simulink subsystem "PowerSystemRef"  (R2024b)
settings: Solver=VariableStepAuto  StartTime=0.0  StopTime=10.0  RelTol=1e-3
undefined symbols (not defined in the file): ess, geom, mot, mot2, mot3, mot4, propel, propel2, propel3, propel4, pxf_diagram_options, SimIn, tc, tc2, tc3, tc4
libraries: simulink x10, slpidlib x5
(part 4 of 10)

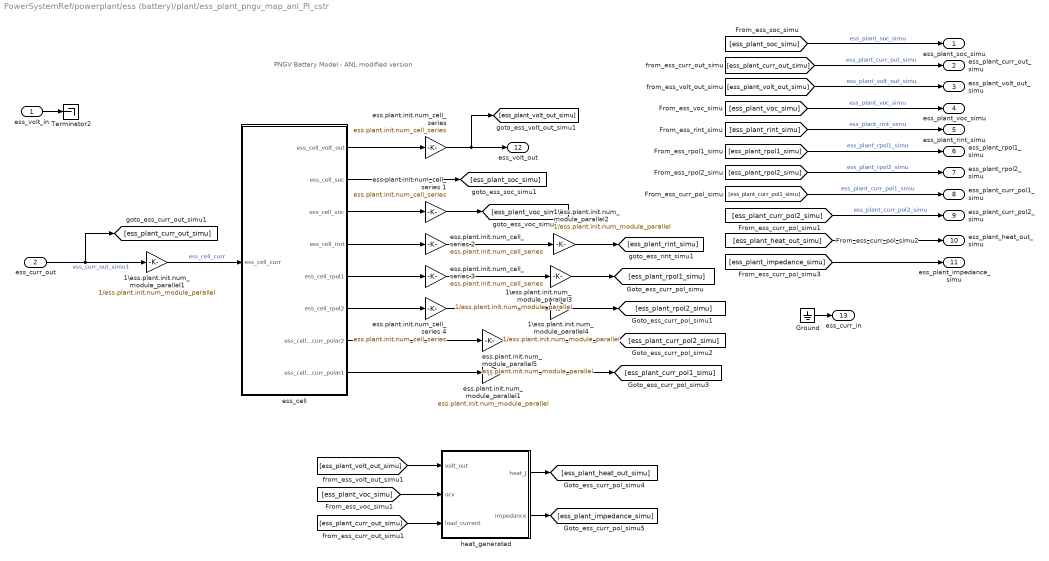
== system PowerSystemRef/powerplant/ess (battery)/plant/ess_plant_pngv_map_anl_PI_cstr ==
  note: PNGV Battery Model - ANL modified version
  ess_volt_in : Inport
  ess_curr_out : Inport  Port=2
  1\ess.plant.init.num_module_parallel{1..4} (4 alike) : Gain  Gain=1/ess.plant.init.num_module_parallel
  Ground : Ground
  Terminator2 : Terminator
  ess.plant.init.num_cell_series {,1..4} (5 alike) : Gain  Gain=ess.plant.init.num_cell_series
  ess.plant.init.num_module_parallel1 : Gain  Gain=ess.plant.init.num_module_parallel
  ess.plant.init.num_module_parallel5 : Gain  Gain=ess.plant.init.num_module_parallel
  ess_cell : Subsystem
  heat_generated : Subsystem
  ess_plant_soc_simu : Outport
  ess_plant_curr_out_simu : Outport  Port=2
  ess_plant_volt_out_simu : Outport  Port=3
  ess_plant_voc_simu : Outport  Port=4
  ess_plant_rint_simu : Outport  Port=5
  ess_plant_rpol1_simu : Outport  Port=6
  ess_plant_rpol2_simu : Outport  Port=7
  ess_plant_curr_pol1_simu : Outport  Port=8
  ess_plant_curr_pol2_simu : Outport  Port=9
  ess_plant_heat_out_simu : Outport  Port=10
  ess_plant_impedance_simu : Outport  Port=11
  ess_volt_out : Outport  Port=12
  ess_curr_in : Outport  Port=13
  wires:
  [ess_plant_impedance_simu] -> ess_plant_impedance_simu/1
  heat_generated/2(impedance) -> [ess_plant_impedance_simu]
  [ess_plant_heat_out_simu] -> ess_plant_heat_out_simu/1
  heat_generated/1(heat_J) -> [ess_plant_heat_out_simu]
  [ess_plant_curr_out_simu] -> heat_generated/3(load_current)
  [ess_plant_voc_simu] -> heat_generated/2(ocv)
  [ess_plant_volt_out_simu] -> heat_generated/1(volt_out)
  ess.plant.init.num_module_parallel1/1 -> [ess_plant_curr_pol1_simu]
  ess.plant.init.num_module_parallel5/1 -> [ess_plant_curr_pol2_simu]
  ess_cell/7(ess_cell_curr_polar2) -> ess.plant.init.num_module_parallel5/1
  ess_cell/8(ess_cell_curr_polar1) -> ess.plant.init.num_module_parallel1/1
  1\ess.plant.init.num_module_parallel4/1 -> [ess_plant_rpol2_simu]
  ess.plant.init.num_cell_series 4/1 -> 1\ess.plant.init.num_module_parallel4/1
  1\ess.plant.init.num_module_parallel3/1 -> [ess_plant_rpol1_simu]
  ess.plant.init.num_cell_series 3/1 -> 1\ess.plant.init.num_module_parallel3/1
  ess_cell/6(ess_cell_rpol2) -> ess.plant.init.num_cell_series 4/1
  ess_cell/5(ess_cell_rpol1) -> ess.plant.init.num_cell_series 3/1
  ess_cell/2(ess_cell_soc) -> [ess_plant_soc_simu]
  ess_cell/4(ess_cell_rint) -> ess.plant.init.num_cell_series 2/1
  ess_cell/3(ess_cell_voc) -> ess.plant.init.num_cell_series 1/1
  ess_curr_out/1 -> [ess_plant_curr_out_simu], 1\ess.plant.init.num_module_parallel1/1  "ess_curr_out_simu1"
  1\ess.plant.init.num_module_parallel2/1 -> [ess_plant_rint_simu]
  ess.plant.init.num_cell_series 1/1 -> [ess_plant_voc_simu]
  ess.plant.init.num_cell_series 2/1 -> 1\ess.plant.init.num_module_parallel2/1
  "ess.plant.init.num_cell_series "/1 -> ess_volt_out/1, [ess_plant_volt_out_simu]
  1\ess.plant.init.num_module_parallel1/1 -> ess_cell/1(ess_cell_curr)  "ess_cell_curr"
  ess_cell/1(ess_cell_volt_out) -> "ess.plant.init.num_cell_series "/1
  [ess_plant_curr_pol2_simu] -> ess_plant_curr_pol2_simu/1  "ess_plant_curr_pol2_simu"
  [ess_plant_curr_pol1_simu] -> ess_plant_curr_pol1_simu/1  "ess_plant_curr_pol1_simu"
  [ess_plant_rpol2_simu] -> ess_plant_rpol2_simu/1  "ess_plant_rpol2_simu"
  [ess_plant_rpol1_simu] -> ess_plant_rpol1_simu/1  "ess_plant_rpol1_simu"
  [ess_plant_rint_simu] -> ess_plant_rint_simu/1  "ess_plant_rint_simu"
  [ess_plant_voc_simu] -> ess_plant_voc_simu/1  "ess_plant_voc_simu"
  [ess_plant_volt_out_simu] -> ess_plant_volt_out_simu/1  "ess_plant_volt_out_simu"
  [ess_plant_curr_out_simu] -> ess_plant_curr_out_simu/1  "ess_plant_curr_out_simu"
  [ess_plant_soc_simu] -> ess_plant_soc_simu/1  "ess_plant_soc_simu"
  ess_volt_in/1 -> Terminator2/1
  Ground/1 -> ess_curr_in/1

== system PowerSystemRef/powerplant/ess (battery)/plant/parameter_out ==
  inport-ess_plant_soc_simu : Inport
  inport-ess_plant_curr_out_simu : Inport  Port=2
  inport-ess_plant_volt_out_simu : Inport  Port=3
  inport-ess_plant_voc_simu : Inport  Port=4
  inport-ess_plant_rint_simu : Inport  Port=5
  inport-ess_plant_rpol1_simu : Inport  Port=6
  inport-ess_plant_rpol2_simu : Inport  Port=7
  inport-ess_plant_curr_pol1_simu : Inport  Port=8
  inport-ess_plant_curr_pol2_simu : Inport  Port=9
  inport-ess_plant_heat_out_simu : Inport  Port=10
  inport-ess_plant_impedance_simu : Inport  Port=11
  Ground_1 : Ground
  Toworkspace-ess_plant_curr_out_simu : ToWorkspace  VariableName=ess_plant_curr_out_simu  SampleTime=pxf_diagram_options.workspace_sample_time
      settings: Decimation=pxf_diagram_options.decimation
  Toworkspace-ess_plant_curr_pol1_simu : ToWorkspace  VariableName=ess_plant_curr_pol1_simu  SampleTime=pxf_diagram_options.workspace_sample_time
      settings: Decimation=pxf_diagram_options.decimation
  Toworkspace-ess_plant_curr_pol2_simu : ToWorkspace  VariableName=ess_plant_curr_pol2_simu  SampleTime=pxf_diagram_options.workspace_sample_time
      settings: Decimation=pxf_diagram_options.decimation
  Toworkspace-ess_plant_heat_out_simu : ToWorkspace  VariableName=ess_plant_heat_out_simu  SampleTime=pxf_diagram_options.workspace_sample_time
      settings: Decimation=pxf_diagram_options.decimation
  Toworkspace-ess_plant_impedance_simu : ToWorkspace  VariableName=ess_plant_impedance_simu  SampleTime=pxf_diagram_options.workspace_sample_time
      settings: Decimation=pxf_diagram_options.decimation
  Toworkspace-ess_plant_rint_simu : ToWorkspace  VariableName=ess_plant_rint_simu  SampleTime=pxf_diagram_options.workspace_sample_time
      settings: Decimation=pxf_diagram_options.decimation
  Toworkspace-ess_plant_rpol1_simu : ToWorkspace  VariableName=ess_plant_rpol1_simu  SampleTime=pxf_diagram_options.workspace_sample_time
      settings: Decimation=pxf_diagram_options.decimation
  Toworkspace-ess_plant_rpol2_simu : ToWorkspace  VariableName=ess_plant_rpol2_simu  SampleTime=pxf_diagram_options.workspace_sample_time
      settings: Decimation=pxf_diagram_options.decimation
  Toworkspace-ess_plant_soc_simu : ToWorkspace  VariableName=ess_plant_soc_simu  SampleTime=pxf_diagram_options.workspace_sample_time
      settings: Decimation=pxf_diagram_options.decimation
  Toworkspace-ess_plant_voc_simu : ToWorkspace  VariableName=ess_plant_voc_simu  SampleTime=pxf_diagram_options.workspace_sample_time
      settings: Decimation=pxf_diagram_options.decimation
  Toworkspace-ess_plant_volt_out_simu : ToWorkspace  VariableName=ess_plant_volt_out_simu  SampleTime=pxf_diagram_options.workspace_sample_time
      settings: Decimation=pxf_diagram_options.decimation
  create_system_info_bus : BusCreator  Inputs=3
  outport-system_info_bus : Outport
  outport-plant_bus : Outport  Port=2
  wires:
  create_system_info_bus/1 -> outport-system_info_bus/1
  inport-ess_plant_soc_simu/1 -> create_system_info_bus/1, Toworkspace-ess_plant_soc_simu/1  "ess_plant_soc_simu"
  inport-ess_plant_heat_out_simu/1 -> Toworkspace-ess_plant_heat_out_simu/1
  inport-ess_plant_impedance_simu/1 -> Toworkspace-ess_plant_impedance_simu/1
  inport-ess_plant_curr_out_simu/1 -> create_system_info_bus/2, Toworkspace-ess_plant_curr_out_simu/1  "ess_plant_curr_out_simu"
  inport-ess_plant_volt_out_simu/1 -> create_system_info_bus/3, Toworkspace-ess_plant_volt_out_simu/1  "ess_plant_volt_out_simu"
  inport-ess_plant_voc_simu/1 -> Toworkspace-ess_plant_voc_simu/1
  inport-ess_plant_rint_simu/1 -> Toworkspace-ess_plant_rint_simu/1
  inport-ess_plant_rpol1_simu/1 -> Toworkspace-ess_plant_rpol1_simu/1
  inport-ess_plant_rpol2_simu/1 -> Toworkspace-ess_plant_rpol2_simu/1
  inport-ess_plant_curr_pol1_simu/1 -> Toworkspace-ess_plant_curr_pol1_simu/1
  inport-ess_plant_curr_pol2_simu/1 -> Toworkspace-ess_plant_curr_pol2_simu/1
  Ground_1/1 -> outport-plant_bus/1

== system PowerSystemRef/powerplant/ess (battery)/plant/parameter_selection ==

== system PowerSystemRef/powerplant/ess (battery)1/ctrl/ess_ctrl_pngv_map_anl_PI_cstr ==
  ess_volt_out : Inport
  ess_curr_out : Inport  Port=2
  ess_soc : Inport  Port=3
  Demux : Demux  Outputs=3
  Demux1 : Demux  Outputs=3
  PI controller for maximal charge power and current1 : Subsystem
  PI controller for maximal discharge power and current1 : Subsystem
  mux1 : Mux  Inputs=3
  ess_ctrl_pwr_max_pro_simu : Outport
  ess_ctrl_pwr_max_reg_simu : Outport  Port=2
  ess_ctrl_curr_max_pro_simu : Outport  Port=3
  ess_ctrl_curr_max_reg_simu : Outport  Port=4
  wires:
  [ess_ctrl_pwr_max_reg_simu] -> ess_ctrl_pwr_max_reg_simu/1  "ess_ctrl_pwr_max_reg_simu"
  [ess_ctrl_pwr_max_pro_simu] -> ess_ctrl_pwr_max_pro_simu/1  "ess_ctrl_pwr_max_pro_simu"
  [ess_ctrl_curr_max_pro_simu] -> ess_ctrl_curr_max_pro_simu/1  "ess_ctrl_curr_max_pro_simu"
  [ess_ctrl_curr_max_reg_simu] -> ess_ctrl_curr_max_reg_simu/1  "ess_ctrl_curr_max_reg_simu"
  PI controller for maximal discharge power and current1/1(Curr_max_prop) -> [ess_ctrl_curr_max_pro_simu]
  PI controller for maximal charge power and current1/2(Curr_max_reg) -> [ess_ctrl_curr_max_reg_simu]
  ess_volt_out/1 -> mux1/1  "ess_plant_volt_out_simu"
  mux1/1 -> Demux/1, Demux1/1
  PI controller for maximal discharge power and current1/2(Pwr_max_prop) -> [ess_ctrl_pwr_max_pro_simu]
  PI controller for maximal charge power and current1/1(Pwr_max_reg) -> [ess_ctrl_pwr_max_reg_simu]
  Demux/1 -> PI controller for maximal discharge power and current1/1(ess voltage)
  Demux/2 -> PI controller for maximal discharge power and current1/2(ess curr)
  Demux/3 -> PI controller for maximal discharge power and current1/3(SOC)
  Demux1/1 -> PI controller for maximal charge power and current1/1(ess voltage)
  Demux1/2 -> PI controller for maximal charge power and current1/2(ess curr)
  Demux1/3 -> PI controller for maximal charge power and current1/3(SOC)
  ess_curr_out/1 -> mux1/2  "ess_plant_curr_out_simu"
  ess_soc/1 -> mux1/3  "ess_plant_soc_simu"

== system PowerSystemRef/powerplant/ess (battery)1/ctrl/parameter_out ==
  inport-ess_ctrl_pwr_max_pro_simu : Inport
  inport-ess_ctrl_pwr_max_reg_simu : Inport  Port=2
  inport-ess_ctrl_curr_max_pro_simu : Inport  Port=3
  inport-ess_ctrl_curr_max_reg_simu : Inport  Port=4
  Ground_1 : Ground
  Toworkspace-ess_ctrl_curr_max_pro_simu : ToWorkspace  VariableName=ess_ctrl_curr_max_pro_simu  SampleTime=pxf_diagram_options.workspace_sample_time
      settings: Decimation=pxf_diagram_options.decimation
  Toworkspace-ess_ctrl_curr_max_reg_simu : ToWorkspace  VariableName=ess_ctrl_curr_max_reg_simu  SampleTime=pxf_diagram_options.workspace_sample_time
      settings: Decimation=pxf_diagram_options.decimation
  Toworkspace-ess_ctrl_pwr_max_pro_simu : ToWorkspace  VariableName=ess_ctrl_pwr_max_pro_simu  SampleTime=pxf_diagram_options.workspace_sample_time
      settings: Decimation=pxf_diagram_options.decimation
  Toworkspace-ess_ctrl_pwr_max_reg_simu : ToWorkspace  VariableName=ess_ctrl_pwr_max_reg_simu  SampleTime=pxf_diagram_options.workspace_sample_time
      settings: Decimation=pxf_diagram_options.decimation
  create_system_info_bus : BusCreator  Inputs=1
  outport-system_info_bus : Outport
  outport-ctrl_bus : Outport  Port=2
  wires:
  Ground_1/1 -> outport-ctrl_bus/1
  inport-ess_ctrl_curr_max_reg_simu/1 -> Toworkspace-ess_ctrl_curr_max_reg_simu/1
  inport-ess_ctrl_curr_max_pro_simu/1 -> Toworkspace-ess_ctrl_curr_max_pro_simu/1
  inport-ess_ctrl_pwr_max_reg_simu/1 -> Toworkspace-ess_ctrl_pwr_max_reg_simu/1
  inport-ess_ctrl_pwr_max_pro_simu/1 -> Toworkspace-ess_ctrl_pwr_max_pro_simu/1, create_system_info_bus/1  "ess_ctrl_pwr_max_pro_simu"
  create_system_info_bus/1 -> outport-system_info_bus/1

== system PowerSystemRef/powerplant/ess (battery)1/ctrl/parameter_selection ==
  inport-main_info_bus-1 : Inport
  select_main_info_bus : BusSelector  OutputSignals=apa_info_bus.powerplant_info_bus.ess.plant.ess_plant_volt_out_simu,apa_info_bus.powerplant_info_bus.ess.plant.ess_plant_curr_out_simu,apa_info_bus.powerplant_info_bus.ess.plant.ess_plant_soc_simu
  outport-ess_plant_volt_out_simu-1 : Outport
  outport-ess_plant_curr_out_simu-2 : Outport  Port=2
  outport-ess_plant_soc_simu-3 : Outport  Port=3
  wires:
  select_main_info_bus/3 -> outport-ess_plant_soc_simu-3/1  "<ess_plant_soc_simu>"
  select_main_info_bus/2 -> outport-ess_plant_curr_out_simu-2/1  "<ess_plant_curr_out_simu>"
  select_main_info_bus/1 -> outport-ess_plant_volt_out_simu-1/1  "<ess_plant_volt_out_simu>"
  inport-main_info_bus-1/1 -> select_main_info_bus/1

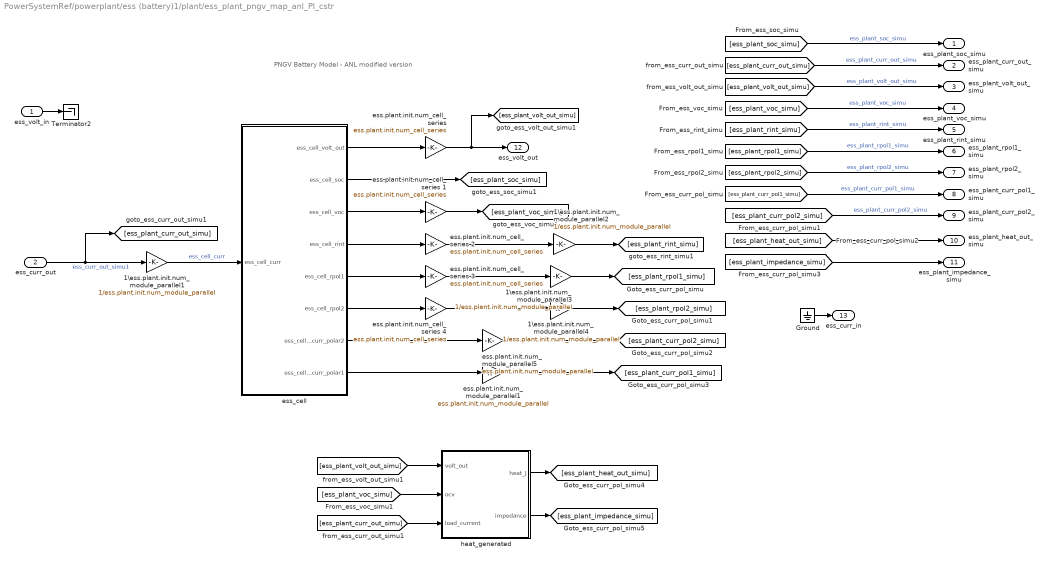
== system PowerSystemRef/powerplant/ess (battery)1/plant/ess_plant_pngv_map_anl_PI_cstr ==
  note: PNGV Battery Model - ANL modified version
  ess_volt_in : Inport
  ess_curr_out : Inport  Port=2
  1\ess.plant.init.num_module_parallel{1..4} (4 alike) : Gain  Gain=1/ess.plant.init.num_module_parallel
  Ground : Ground
  Terminator2 : Terminator
  ess.plant.init.num_cell_series {,1..4} (5 alike) : Gain  Gain=ess.plant.init.num_cell_series
  ess.plant.init.num_module_parallel1 : Gain  Gain=ess.plant.init.num_module_parallel
  ess.plant.init.num_module_parallel5 : Gain  Gain=ess.plant.init.num_module_parallel
  ess_cell : Subsystem
  heat_generated : Subsystem
  ess_plant_soc_simu : Outport
  ess_plant_curr_out_simu : Outport  Port=2
  ess_plant_volt_out_simu : Outport  Port=3
  ess_plant_voc_simu : Outport  Port=4
  ess_plant_rint_simu : Outport  Port=5
  ess_plant_rpol1_simu : Outport  Port=6
  ess_plant_rpol2_simu : Outport  Port=7
  ess_plant_curr_pol1_simu : Outport  Port=8
  ess_plant_curr_pol2_simu : Outport  Port=9
  ess_plant_heat_out_simu : Outport  Port=10
  ess_plant_impedance_simu : Outport  Port=11
  ess_volt_out : Outport  Port=12
  ess_curr_in : Outport  Port=13
  wires:
  Ground/1 -> ess_curr_in/1
  ess_volt_in/1 -> Terminator2/1
  [ess_plant_soc_simu] -> ess_plant_soc_simu/1  "ess_plant_soc_simu"
  [ess_plant_curr_out_simu] -> ess_plant_curr_out_simu/1  "ess_plant_curr_out_simu"
  [ess_plant_volt_out_simu] -> ess_plant_volt_out_simu/1  "ess_plant_volt_out_simu"
  [ess_plant_voc_simu] -> ess_plant_voc_simu/1  "ess_plant_voc_simu"
  [ess_plant_rint_simu] -> ess_plant_rint_simu/1  "ess_plant_rint_simu"
  [ess_plant_rpol1_simu] -> ess_plant_rpol1_simu/1  "ess_plant_rpol1_simu"
  [ess_plant_rpol2_simu] -> ess_plant_rpol2_simu/1  "ess_plant_rpol2_simu"
  [ess_plant_curr_pol1_simu] -> ess_plant_curr_pol1_simu/1  "ess_plant_curr_pol1_simu"
  [ess_plant_curr_pol2_simu] -> ess_plant_curr_pol2_simu/1  "ess_plant_curr_pol2_simu"
  ess_cell/1(ess_cell_volt_out) -> "ess.plant.init.num_cell_series "/1
  1\ess.plant.init.num_module_parallel1/1 -> ess_cell/1(ess_cell_curr)  "ess_cell_curr"
  "ess.plant.init.num_cell_series "/1 -> [ess_plant_volt_out_simu], ess_volt_out/1
  ess.plant.init.num_cell_series 2/1 -> 1\ess.plant.init.num_module_parallel2/1
  ess.plant.init.num_cell_series 1/1 -> [ess_plant_voc_simu]
  1\ess.plant.init.num_module_parallel2/1 -> [ess_plant_rint_simu]
  ess_curr_out/1 -> 1\ess.plant.init.num_module_parallel1/1, [ess_plant_curr_out_simu]  "ess_curr_out_simu1"
  ess_cell/3(ess_cell_voc) -> ess.plant.init.num_cell_series 1/1
  ess_cell/4(ess_cell_rint) -> ess.plant.init.num_cell_series 2/1
  ess_cell/2(ess_cell_soc) -> [ess_plant_soc_simu]
  ess_cell/5(ess_cell_rpol1) -> ess.plant.init.num_cell_series 3/1
  ess_cell/6(ess_cell_rpol2) -> ess.plant.init.num_cell_series 4/1
  ess.plant.init.num_cell_series 3/1 -> 1\ess.plant.init.num_module_parallel3/1
  1\ess.plant.init.num_module_parallel3/1 -> [ess_plant_rpol1_simu]
  ess.plant.init.num_cell_series 4/1 -> 1\ess.plant.init.num_module_parallel4/1
  1\ess.plant.init.num_module_parallel4/1 -> [ess_plant_rpol2_simu]
  ess_cell/8(ess_cell_curr_polar1) -> ess.plant.init.num_module_parallel1/1
  ess_cell/7(ess_cell_curr_polar2) -> ess.plant.init.num_module_parallel5/1
  ess.plant.init.num_module_parallel5/1 -> [ess_plant_curr_pol2_simu]
  ess.plant.init.num_module_parallel1/1 -> [ess_plant_curr_pol1_simu]
  [ess_plant_volt_out_simu] -> heat_generated/1(volt_out)
  [ess_plant_voc_simu] -> heat_generated/2(ocv)
  [ess_plant_curr_out_simu] -> heat_generated/3(load_current)
  heat_generated/1(heat_J) -> [ess_plant_heat_out_simu]
  [ess_plant_heat_out_simu] -> ess_plant_heat_out_simu/1
  heat_generated/2(impedance) -> [ess_plant_impedance_simu]
  [ess_plant_impedance_simu] -> ess_plant_impedance_simu/1

== system PowerSystemRef/powerplant/ess (battery)1/plant/parameter_out ==
  inport-ess_plant_soc_simu : Inport
  inport-ess_plant_curr_out_simu : Inport  Port=2
  inport-ess_plant_volt_out_simu : Inport  Port=3
  inport-ess_plant_voc_simu : Inport  Port=4
  inport-ess_plant_rint_simu : Inport  Port=5
  inport-ess_plant_rpol1_simu : Inport  Port=6
  inport-ess_plant_rpol2_simu : Inport  Port=7
  inport-ess_plant_curr_pol1_simu : Inport  Port=8
  inport-ess_plant_curr_pol2_simu : Inport  Port=9
  inport-ess_plant_heat_out_simu : Inport  Port=10
  inport-ess_plant_impedance_simu : Inport  Port=11
  Ground_1 : Ground
  Toworkspace-ess_plant_curr_out_simu : ToWorkspace  VariableName=ess_plant_curr_out_simu  SampleTime=pxf_diagram_options.workspace_sample_time
      settings: Decimation=pxf_diagram_options.decimation
  Toworkspace-ess_plant_curr_pol1_simu : ToWorkspace  VariableName=ess_plant_curr_pol1_simu  SampleTime=pxf_diagram_options.workspace_sample_time
      settings: Decimation=pxf_diagram_options.decimation
  Toworkspace-ess_plant_curr_pol2_simu : ToWorkspace  VariableName=ess_plant_curr_pol2_simu  SampleTime=pxf_diagram_options.workspace_sample_time
      settings: Decimation=pxf_diagram_options.decimation
  Toworkspace-ess_plant_heat_out_simu : ToWorkspace  VariableName=ess_plant_heat_out_simu  SampleTime=pxf_diagram_options.workspace_sample_time
      settings: Decimation=pxf_diagram_options.decimation
  Toworkspace-ess_plant_impedance_simu : ToWorkspace  VariableName=ess_plant_impedance_simu  SampleTime=pxf_diagram_options.workspace_sample_time
      settings: Decimation=pxf_diagram_options.decimation
  Toworkspace-ess_plant_rint_simu : ToWorkspace  VariableName=ess_plant_rint_simu  SampleTime=pxf_diagram_options.workspace_sample_time
      settings: Decimation=pxf_diagram_options.decimation
  Toworkspace-ess_plant_rpol1_simu : ToWorkspace  VariableName=ess_plant_rpol1_simu  SampleTime=pxf_diagram_options.workspace_sample_time
      settings: Decimation=pxf_diagram_options.decimation
  Toworkspace-ess_plant_rpol2_simu : ToWorkspace  VariableName=ess_plant_rpol2_simu  SampleTime=pxf_diagram_options.workspace_sample_time
      settings: Decimation=pxf_diagram_options.decimation
  Toworkspace-ess_plant_soc_simu : ToWorkspace  VariableName=ess_plant_soc_simu  SampleTime=pxf_diagram_options.workspace_sample_time
      settings: Decimation=pxf_diagram_options.decimation
  Toworkspace-ess_plant_voc_simu : ToWorkspace  VariableName=ess_plant_voc_simu  SampleTime=pxf_diagram_options.workspace_sample_time
      settings: Decimation=pxf_diagram_options.decimation
  Toworkspace-ess_plant_volt_out_simu : ToWorkspace  VariableName=ess_plant_volt_out_simu  SampleTime=pxf_diagram_options.workspace_sample_time
      settings: Decimation=pxf_diagram_options.decimation
  create_system_info_bus : BusCreator  Inputs=3
  outport-system_info_bus : Outport
  outport-plant_bus : Outport  Port=2
  wires:
  Ground_1/1 -> outport-plant_bus/1
  inport-ess_plant_curr_pol2_simu/1 -> Toworkspace-ess_plant_curr_pol2_simu/1
  inport-ess_plant_curr_pol1_simu/1 -> Toworkspace-ess_plant_curr_pol1_simu/1
  inport-ess_plant_rpol2_simu/1 -> Toworkspace-ess_plant_rpol2_simu/1
  inport-ess_plant_rpol1_simu/1 -> Toworkspace-ess_plant_rpol1_simu/1
  inport-ess_plant_rint_simu/1 -> Toworkspace-ess_plant_rint_simu/1
  inport-ess_plant_voc_simu/1 -> Toworkspace-ess_plant_voc_simu/1
  inport-ess_plant_volt_out_simu/1 -> Toworkspace-ess_plant_volt_out_simu/1, create_system_info_bus/3  "ess_plant_volt_out_simu"
  inport-ess_plant_curr_out_simu/1 -> Toworkspace-ess_plant_curr_out_simu/1, create_system_info_bus/2  "ess_plant_curr_out_simu"
  inport-ess_plant_impedance_simu/1 -> Toworkspace-ess_plant_impedance_simu/1
  inport-ess_plant_heat_out_simu/1 -> Toworkspace-ess_plant_heat_out_simu/1
  inport-ess_plant_soc_simu/1 -> Toworkspace-ess_plant_soc_simu/1, create_system_info_bus/1  "ess_plant_soc_simu"
  create_system_info_bus/1 -> outport-system_info_bus/1

== system PowerSystemRef/powerplant/ess (battery)1/plant/parameter_selection ==

== system PowerSystemRef/powerplant/mot/ctrl/cmd ==
  inport-main_info_bus-1 : Inport
  aInport--2 : Inport  Port=2
  aInport--3 : Inport  Port=3
  aInport--4 : Inport  Port=4
  Terminator_1 : Terminator
  Terminator_2 : Terminator
  Terminator_3 : Terminator
  mot_ctrl_cmd_map_Pelec_funTW_volt_in : Subsystem
  parameter_out : Subsystem
  parameter_selection : Subsystem
  outport-system_info_bus : Outport
  wires:
  inport-main_info_bus-1/1 -> parameter_selection/1(inport-main_info_bus-1)
  parameter_out/1(outport-system_info_bus) -> outport-system_info_bus/1
  mot_ctrl_cmd_map_Pelec_funTW_volt_in/1(mot_ctrl_cmd_simu) -> parameter_out/1(inport-mot_ctrl_cmd_simu)
  parameter_selection/1(outport-mot_plant_spd_out_simu-1) -> mot_ctrl_cmd_map_Pelec_funTW_volt_in/1(mot_plant_spd_out_simu)
  parameter_selection/2(outport-mot_ctrl_trs_trq_simu-2) -> mot_ctrl_cmd_map_Pelec_funTW_volt_in/2(mot_ctrl_trs_trq_simu)
  parameter_selection/3(outport-mot_ctrl_cstr_trq_max_pos_simu-3) -> mot_ctrl_cmd_map_Pelec_funTW_volt_in/3(mot_ctrl_cstr_trq_max_pos_simu)
  parameter_selection/4(outport-mot_ctrl_cstr_trq_max_neg_simu-4) -> mot_ctrl_cmd_map_Pelec_funTW_volt_in/4(mot_ctrl_cstr_trq_max_neg_simu)
  aInport--2/1 -> Terminator_1/1
  aInport--3/1 -> Terminator_2/1
  aInport--4/1 -> Terminator_3/1

== system PowerSystemRef/powerplant/mot/ctrl/cstr ==
  inport-main_info_bus-1 : Inport
  aInport--2 : Inport  Port=2
  aInport--3 : Inport  Port=3
  Terminator_1 : Terminator
  Terminator_2 : Terminator
  mot_ctrl_cstr_map_Pelec_funTW_volt_in : Subsystem
  parameter_out : Subsystem
  parameter_selection : Subsystem
  outport-system_info_bus : Outport
  outport-cstr_bus : Outport  Port=2
  wires:
  inport-main_info_bus-1/1 -> parameter_selection/1(inport-main_info_bus-1)
  parameter_out/1(outport-system_info_bus) -> outport-system_info_bus/1
  parameter_out/2(outport-cstr_bus) -> outport-cstr_bus/1
  mot_ctrl_cstr_map_Pelec_funTW_volt_in/1(mot_ctrl_cstr_trq_pk_pos_simu) -> parameter_out/1(inport-mot_ctrl_cstr_trq_pk_pos_simu)
  mot_ctrl_cstr_map_Pelec_funTW_volt_in/2(mot_ctrl_cstr_trq_max_pos_simu) -> parameter_out/2(inport-mot_ctrl_cstr_trq_max_pos_simu)
  mot_ctrl_cstr_map_Pelec_funTW_volt_in/3(mot_ctrl_cstr_trq_pk_neg_simu) -> parameter_out/3(inport-mot_ctrl_cstr_trq_pk_neg_simu)
  mot_ctrl_cstr_map_Pelec_funTW_volt_in/4(mot_ctrl_cstr_trq_max_neg_simu) -> parameter_out/4(inport-mot_ctrl_cstr_trq_max_neg_simu)
  mot_ctrl_cstr_map_Pelec_funTW_volt_in/5(mot_ctrl_cstr_trq_cont_pos_simu) -> parameter_out/5(inport-mot_ctrl_cstr_trq_cont_pos_simu)
  mot_ctrl_cstr_map_Pelec_funTW_volt_in/6(mot_ctrl_cstr_trq_cont_neg_simu) -> parameter_out/6(inport-mot_ctrl_cstr_trq_cont_neg_simu)
  mot_ctrl_cstr_map_Pelec_funTW_volt_in/7(mot_ctrl_cstr_temp_coeff_simu) -> parameter_out/7(inport-mot_ctrl_cstr_temp_coeff_simu)
  parameter_selection/1(outport-mot_plant_spd_out_simu-1) -> mot_ctrl_cstr_map_Pelec_funTW_volt_in/1(mot_plant_spd_out_simu)
  parameter_selection/2(outport-mot_plant_temp_coeff_simu-2) -> mot_ctrl_cstr_map_Pelec_funTW_volt_in/2(mot_plant_temp_coeff_simu)
  aInport--2/1 -> Terminator_1/1
  aInport--3/1 -> Terminator_2/1

== system PowerSystemRef/powerplant/mot/ctrl/dmd ==
  inport-main_info_bus-1 : Inport
  aInport--2 : Inport  Port=2
  Terminator_1 : Terminator
  mot_ctrl_dmd_uas : Subsystem
  parameter_out : Subsystem
  parameter_selection : Subsystem
  outport-system_info_bus : Outport
  outport-dmd_bus : Outport  Port=2
  wires:
  inport-main_info_bus-1/1 -> parameter_selection/1(inport-main_info_bus-1)
  parameter_out/1(outport-system_info_bus) -> outport-system_info_bus/1
  parameter_out/2(outport-dmd_bus) -> outport-dmd_bus/1
  mot_ctrl_dmd_uas/1(mot_ctrl_trs_trq_simu) -> parameter_out/1(inport-mot_ctrl_trs_trq_simu)
  mot_ctrl_dmd_uas/2(mot_ctrl_ratedpwr_simu) -> parameter_out/2(inport-mot_ctrl_ratedpwr_simu)
  parameter_selection/1(outport-apc_ctrl_dt1_simu-1) -> mot_ctrl_dmd_uas/1(apc_ctrl_dt_simu)
  parameter_selection/2(outport-env_plant_density_simu-2) -> mot_ctrl_dmd_uas/2(env_plant_density_simu)
  parameter_selection/3(outport-ess_ctrl_pwr_max_pro_simu-3) -> mot_ctrl_dmd_uas/3(ess_ctrl_pwr_max_pro_simu)
  parameter_selection/4(outport-propel_plant_speed_simu-4) -> mot_ctrl_dmd_uas/4(propel_plant_speed_simu)
  parameter_selection/5(outport-tc_plant_spd_in_simu-5) -> mot_ctrl_dmd_uas/5(tc_plant_spd_in_simu)
  aInport--2/1 -> Terminator_1/1

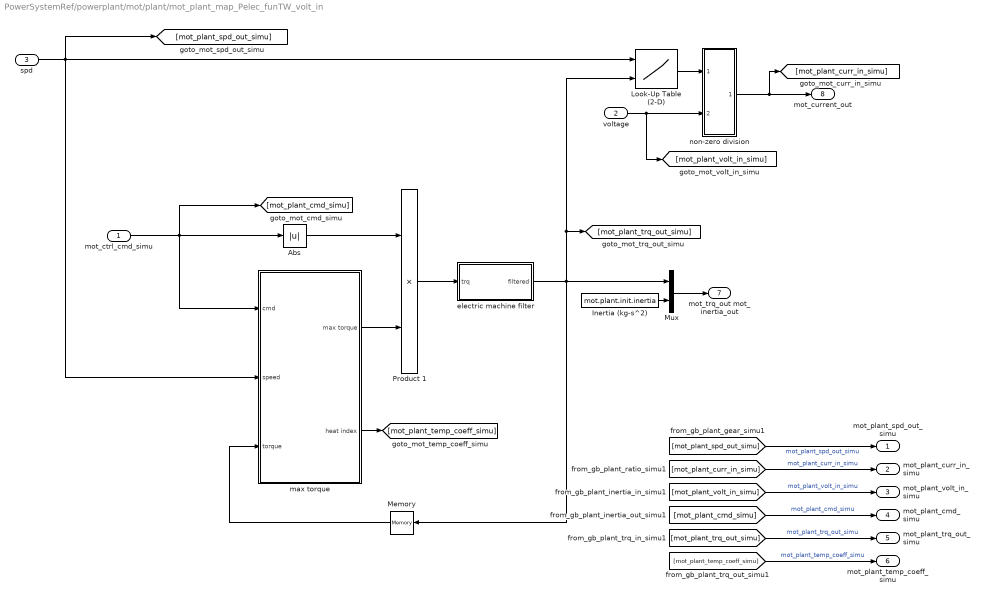
== system PowerSystemRef/powerplant/mot/plant/mot_plant_map_Pelec_funTW_volt_in ==
  mot_ctrl_cmd_simu : Inport
  voltage : Inport  Port=2
  spd : Inport  Port=3
  Abs : Abs
  Inertia (kg-s^2) : Constant  Value=mot.plant.init.inertia
  Look-Up Table (2-D) : Lookup2D  RowIndex=mot.plant.calc.pwr_elec.idx1_spd  ColumnIndex=mot.plant.calc.pwr_elec.idx2_trq  Table=mot.plant.calc.pwr_elec.map
  Memory : Memory
  Mux : Mux  Inputs=2
  Product 1 : Product  InputSameDT=on  SaturateOnIntegerOverflow=on  OutDataTypeStr=Inherit: Same as first input
  electric machine filter : Subsystem
  "max torque " : Subsystem
  non-zero division : Subsystem
      mask Display: disp('divider \n I1/I2')
  mot_plant_spd_out_simu : Outport
  mot_plant_curr_in_simu : Outport  Port=2
  mot_plant_volt_in_simu : Outport  Port=3
  mot_plant_cmd_simu : Outport  Port=4
  mot_plant_trq_out_simu : Outport  Port=5
  mot_plant_temp_coeff_simu : Outport  Port=6
  mot_trq_out mot_inertia_out : Outport  Port=7
  mot_current_out : Outport  Port=8
  wires:
  Look-Up Table (2-D)/1 -> non-zero division/1(In1)
  [mot_plant_temp_coeff_simu] -> mot_plant_temp_coeff_simu/1  "mot_plant_temp_coeff_simu"
  [mot_plant_trq_out_simu] -> mot_plant_trq_out_simu/1  "mot_plant_trq_out_simu"
  [mot_plant_cmd_simu] -> mot_plant_cmd_simu/1  "mot_plant_cmd_simu"
  [mot_plant_volt_in_simu] -> mot_plant_volt_in_simu/1  "mot_plant_volt_in_simu"
  [mot_plant_curr_in_simu] -> mot_plant_curr_in_simu/1  "mot_plant_curr_in_simu"
  [mot_plant_spd_out_simu] -> mot_plant_spd_out_simu/1  "mot_plant_spd_out_simu"
  electric machine filter/1(filtered) -> Mux/1, Memory/1, [mot_plant_trq_out_simu], Look-Up Table (2-D)/2
  "max torque "/1(max torque) -> Product 1/2
  Product 1/1 -> electric machine filter/1(trq)
  Abs/1 -> Product 1/1
  Memory/1 -> "max torque "/3(torque)
  mot_ctrl_cmd_simu/1 -> "max torque "/1(cmd), [mot_plant_cmd_simu], Abs/1
  Inertia (kg-s^2)/1 -> Mux/2
  Mux/1 -> mot_trq_out mot_inertia_out/1
  spd/1 -> [mot_plant_spd_out_simu], "max torque "/2(speed), Look-Up Table (2-D)/1
  "max torque "/2(heat index) -> [mot_plant_temp_coeff_simu]
  non-zero division/1(Out1) -> mot_current_out/1, [mot_plant_curr_in_simu]
  voltage/1 -> non-zero division/2(In2), [mot_plant_volt_in_simu]

== system PowerSystemRef/powerplant/mot/plant/parameter_out ==
  inport-mot_plant_spd_out_simu : Inport
  inport-mot_plant_curr_in_simu : Inport  Port=2
  inport-mot_plant_volt_in_simu : Inport  Port=3
  inport-mot_plant_cmd_simu : Inport  Port=4
  inport-mot_plant_trq_out_simu : Inport  Port=5
  inport-mot_plant_temp_coeff_simu : Inport  Port=6
  Ground_1 : Ground
  Toworkspace-mot_plant_cmd_simu : ToWorkspace  VariableName=mot_plant_cmd_simu  SampleTime=pxf_diagram_options.workspace_sample_time
      settings: Decimation=pxf_diagram_options.decimation
  Toworkspace-mot_plant_curr_in_simu : ToWorkspace  VariableName=mot_plant_curr_in_simu  SampleTime=pxf_diagram_options.workspace_sample_time
      settings: Decimation=pxf_diagram_options.decimation
  Toworkspace-mot_plant_spd_out_simu : ToWorkspace  VariableName=mot_plant_spd_out_simu  SampleTime=pxf_diagram_options.workspace_sample_time
      settings: Decimation=pxf_diagram_options.decimation
  Toworkspace-mot_plant_temp_coeff_simu : ToWorkspace  VariableName=mot_plant_temp_coeff_simu  SampleTime=pxf_diagram_options.workspace_sample_time
      settings: Decimation=pxf_diagram_options.decimation
  Toworkspace-mot_plant_trq_out_simu : ToWorkspace  VariableName=mot_plant_trq_out_simu  SampleTime=pxf_diagram_options.workspace_sample_time
      settings: Decimation=pxf_diagram_options.decimation
  Toworkspace-mot_plant_volt_in_simu : ToWorkspace  VariableName=mot_plant_volt_in_simu  SampleTime=pxf_diagram_options.workspace_sample_time
      settings: Decimation=pxf_diagram_options.decimation
  create_system_info_bus : BusCreator  Inputs=2
  outport-system_info_bus : Outport
  outport-plant_bus : Outport  Port=2
  wires:
  create_system_info_bus/1 -> outport-system_info_bus/1
  inport-mot_plant_spd_out_simu/1 -> create_system_info_bus/1, Toworkspace-mot_plant_spd_out_simu/1  "mot_plant_spd_out_simu"
  inport-mot_plant_curr_in_simu/1 -> Toworkspace-mot_plant_curr_in_simu/1
  inport-mot_plant_volt_in_simu/1 -> Toworkspace-mot_plant_volt_in_simu/1
  inport-mot_plant_cmd_simu/1 -> Toworkspace-mot_plant_cmd_simu/1
  inport-mot_plant_trq_out_simu/1 -> Toworkspace-mot_plant_trq_out_simu/1
  inport-mot_plant_temp_coeff_simu/1 -> create_system_info_bus/2, Toworkspace-mot_plant_temp_coeff_simu/1  "mot_plant_temp_coeff_simu"
  Ground_1/1 -> outport-plant_bus/1

== system PowerSystemRef/powerplant/mot/plant/parameter_selection ==
  Inport_1 : Inport
  inport-ctrl_bus-2 : Inport  Port=2
  Terminator_1 : Terminator
  select_ctrl_bus : BusSelector  OutputSignals=mot_ctrl_cmd_simu
  outport-mot_ctrl_cmd_simu-1 : Outport
  wires:
  inport-ctrl_bus-2/1 -> select_ctrl_bus/1
  select_ctrl_bus/1 -> outport-mot_ctrl_cmd_simu-1/1  "<mot_ctrl_cmd_simu>"
  Inport_1/1 -> Terminator_1/1

== system PowerSystemRef/powerplant/mot2/ctrl/cmd ==
  inport-main_info_bus-1 : Inport
  aInport--2 : Inport  Port=2
  aInport--3 : Inport  Port=3
  aInport--4 : Inport  Port=4
  Terminator_1 : Terminator
  Terminator_2 : Terminator
  Terminator_3 : Terminator
  mot2_ctrl_cmd_map_Pelec_funTW_volt_in : Subsystem
  parameter_out : Subsystem
  parameter_selection : Subsystem
  outport-system_info_bus : Outport
  wires:
  inport-main_info_bus-1/1 -> parameter_selection/1(inport-main_info_bus-1)
  parameter_out/1(outport-system_info_bus) -> outport-system_info_bus/1
  mot2_ctrl_cmd_map_Pelec_funTW_volt_in/1(mot_ctrl_cmd_simu) -> parameter_out/1(inport-mot2_ctrl_cmd_simu)
  parameter_selection/1(outport-mot2_plant_spd_out_simu-1) -> mot2_ctrl_cmd_map_Pelec_funTW_volt_in/1(mot_plant_spd_out_simu)
  parameter_selection/2(outport-mot2_ctrl_trs_trq_simu-2) -> mot2_ctrl_cmd_map_Pelec_funTW_volt_in/2(mot_ctrl_trs_trq_simu)
  parameter_selection/3(outport-mot2_ctrl_cstr_trq_max_pos_simu-3) -> mot2_ctrl_cmd_map_Pelec_funTW_volt_in/3(mot_ctrl_cstr_trq_max_pos_simu)
  parameter_selection/4(outport-mot2_ctrl_cstr_trq_max_neg_simu-4) -> mot2_ctrl_cmd_map_Pelec_funTW_volt_in/4(mot_ctrl_cstr_trq_max_neg_simu)
  aInport--2/1 -> Terminator_1/1
  aInport--3/1 -> Terminator_2/1
  aInport--4/1 -> Terminator_3/1

== system PowerSystemRef/powerplant/mot2/ctrl/cstr ==
  inport-main_info_bus-1 : Inport
  aInport--2 : Inport  Port=2
  aInport--3 : Inport  Port=3
  Terminator_1 : Terminator
  Terminator_2 : Terminator
  mot2_ctrl_cstr_map_Pelec_funTW_volt_in : Subsystem
  parameter_out : Subsystem
  parameter_selection : Subsystem
  outport-system_info_bus : Outport
  outport-cstr_bus : Outport  Port=2
  wires:
  inport-main_info_bus-1/1 -> parameter_selection/1(inport-main_info_bus-1)
  parameter_out/1(outport-system_info_bus) -> outport-system_info_bus/1
  parameter_out/2(outport-cstr_bus) -> outport-cstr_bus/1
  mot2_ctrl_cstr_map_Pelec_funTW_volt_in/1(mot_ctrl_cstr_trq_pk_pos_simu) -> parameter_out/1(inport-mot2_ctrl_cstr_trq_pk_pos_simu)
  mot2_ctrl_cstr_map_Pelec_funTW_volt_in/2(mot_ctrl_cstr_trq_max_pos_simu) -> parameter_out/2(inport-mot2_ctrl_cstr_trq_max_pos_simu)
  mot2_ctrl_cstr_map_Pelec_funTW_volt_in/3(mot_ctrl_cstr_trq_pk_neg_simu) -> parameter_out/3(inport-mot2_ctrl_cstr_trq_pk_neg_simu)
  mot2_ctrl_cstr_map_Pelec_funTW_volt_in/4(mot_ctrl_cstr_trq_max_neg_simu) -> parameter_out/4(inport-mot2_ctrl_cstr_trq_max_neg_simu)
  mot2_ctrl_cstr_map_Pelec_funTW_volt_in/5(mot_ctrl_cstr_trq_cont_pos_simu) -> parameter_out/5(inport-mot2_ctrl_cstr_trq_cont_pos_simu)
  mot2_ctrl_cstr_map_Pelec_funTW_volt_in/6(mot_ctrl_cstr_trq_cont_neg_simu) -> parameter_out/6(inport-mot2_ctrl_cstr_trq_cont_neg_simu)
  mot2_ctrl_cstr_map_Pelec_funTW_volt_in/7(mot_ctrl_cstr_temp_coeff_simu) -> parameter_out/7(inport-mot2_ctrl_cstr_temp_coeff_simu)
  parameter_selection/1(outport-mot2_plant_spd_out_simu-1) -> mot2_ctrl_cstr_map_Pelec_funTW_volt_in/1(mot_plant_spd_out_simu)
  parameter_selection/2(outport-mot2_plant_temp_coeff_simu-2) -> mot2_ctrl_cstr_map_Pelec_funTW_volt_in/2(mot_plant_temp_coeff_simu)
  aInport--2/1 -> Terminator_1/1
  aInport--3/1 -> Terminator_2/1

== system PowerSystemRef/powerplant/mot2/ctrl/dmd ==
  inport-main_info_bus-1 : Inport
  aInport--2 : Inport  Port=2
  Terminator_1 : Terminator
  mot2_ctrl_dmd_uas : Subsystem
  parameter_out : Subsystem
  parameter_selection : Subsystem
  outport-system_info_bus : Outport
  outport-dmd_bus : Outport  Port=2
  wires:
  inport-main_info_bus-1/1 -> parameter_selection/1(inport-main_info_bus-1)
  parameter_out/1(outport-system_info_bus) -> outport-system_info_bus/1
  parameter_out/2(outport-dmd_bus) -> outport-dmd_bus/1
  mot2_ctrl_dmd_uas/1(mot_ctrl_trs_trq_simu) -> parameter_out/1(inport-mot2_ctrl_trs_trq_simu)
  mot2_ctrl_dmd_uas/2(mot_ctrl_ratedpwr_simu) -> parameter_out/2(inport-mot2_ctrl_ratedpwr_simu)
  parameter_selection/1(outport-apc_ctrl_dt2_simu-1) -> mot2_ctrl_dmd_uas/1(apc_ctrl_dt_simu)
  parameter_selection/2(outport-env_plant_density_simu-2) -> mot2_ctrl_dmd_uas/2(env_plant_density_simu)
  parameter_selection/3(outport-ess_ctrl_pwr_max_pro_simu-3) -> mot2_ctrl_dmd_uas/3(ess_ctrl_pwr_max_pro_simu)
  parameter_selection/4(outport-propel2_plant_speed_simu-4) -> mot2_ctrl_dmd_uas/4(propel_plant_speed_simu)
  parameter_selection/5(outport-tc2_plant_spd_in_simu-5) -> mot2_ctrl_dmd_uas/5(tc_plant_spd_in_simu)
  aInport--2/1 -> Terminator_1/1

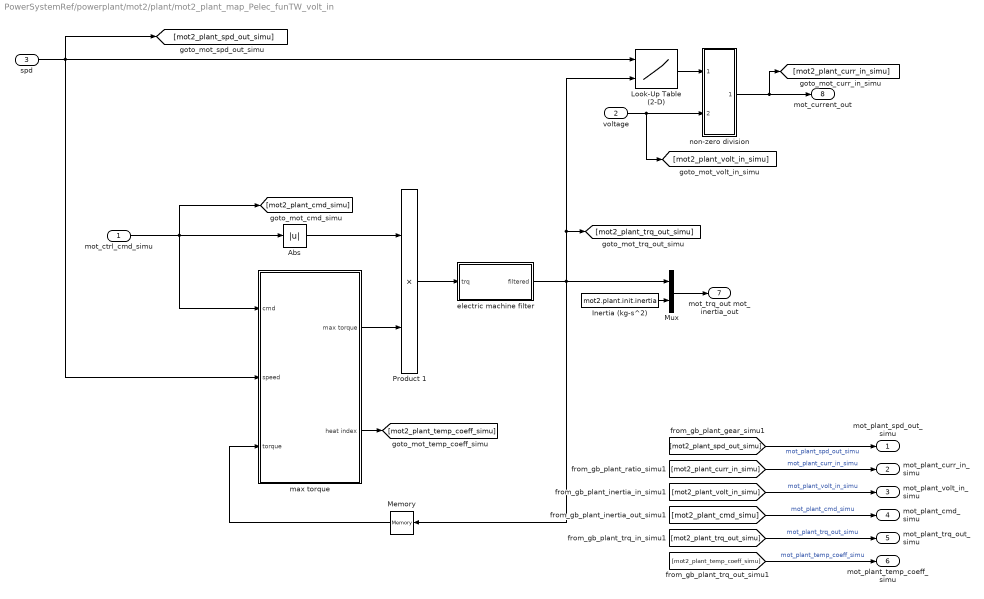
== system PowerSystemRef/powerplant/mot2/plant/mot2_plant_map_Pelec_funTW_volt_in ==
  mot_ctrl_cmd_simu : Inport
  voltage : Inport  Port=2
  spd : Inport  Port=3
  Abs : Abs
  Inertia (kg-s^2) : Constant  Value=mot2.plant.init.inertia
  Look-Up Table (2-D) : Lookup2D  RowIndex=mot2.plant.calc.pwr_elec.idx1_spd  ColumnIndex=mot2.plant.calc.pwr_elec.idx2_trq  Table=mot2.plant.calc.pwr_elec.map
  Memory : Memory
  Mux : Mux  Inputs=2
  Product 1 : Product  InputSameDT=on  SaturateOnIntegerOverflow=on  OutDataTypeStr=Inherit: Same as first input
  electric machine filter : Subsystem
  "max torque " : Subsystem
  non-zero division : Subsystem
      mask Display: disp('divider \n I1/I2')
  mot_plant_spd_out_simu : Outport
  mot_plant_curr_in_simu : Outport  Port=2
  mot_plant_volt_in_simu : Outport  Port=3
  mot_plant_cmd_simu : Outport  Port=4
  mot_plant_trq_out_simu : Outport  Port=5
  mot_plant_temp_coeff_simu : Outport  Port=6
  mot_trq_out mot_inertia_out : Outport  Port=7
  mot_current_out : Outport  Port=8
  wires:
  Look-Up Table (2-D)/1 -> non-zero division/1(In1)
  [mot2_plant_temp_coeff_simu] -> mot_plant_temp_coeff_simu/1  "mot_plant_temp_coeff_simu"
  [mot2_plant_trq_out_simu] -> mot_plant_trq_out_simu/1  "mot_plant_trq_out_simu"
  [mot2_plant_cmd_simu] -> mot_plant_cmd_simu/1  "mot_plant_cmd_simu"
  [mot2_plant_volt_in_simu] -> mot_plant_volt_in_simu/1  "mot_plant_volt_in_simu"
  [mot2_plant_curr_in_simu] -> mot_plant_curr_in_simu/1  "mot_plant_curr_in_simu"
  [mot2_plant_spd_out_simu] -> mot_plant_spd_out_simu/1  "mot_plant_spd_out_simu"
  electric machine filter/1(filtered) -> Mux/1, Memory/1, [mot2_plant_trq_out_simu], Look-Up Table (2-D)/2
  "max torque "/1(max torque) -> Product 1/2
  Product 1/1 -> electric machine filter/1(trq)
  Abs/1 -> Product 1/1
  Memory/1 -> "max torque "/3(torque)
  mot_ctrl_cmd_simu/1 -> "max torque "/1(cmd), [mot2_plant_cmd_simu], Abs/1
  Inertia (kg-s^2)/1 -> Mux/2
  Mux/1 -> mot_trq_out mot_inertia_out/1
  spd/1 -> [mot2_plant_spd_out_simu], "max torque "/2(speed), Look-Up Table (2-D)/1
  "max torque "/2(heat index) -> [mot2_plant_temp_coeff_simu]
  non-zero division/1(Out1) -> mot_current_out/1, [mot2_plant_curr_in_simu]
  voltage/1 -> non-zero division/2(In2), [mot2_plant_volt_in_simu]

== system PowerSystemRef/powerplant/mot2/plant/parameter_out ==
  inport-mot2_plant_spd_out_simu : Inport
  inport-mot2_plant_curr_in_simu : Inport  Port=2
  inport-mot2_plant_volt_in_simu : Inport  Port=3
  inport-mot2_plant_cmd_simu : Inport  Port=4
  inport-mot2_plant_trq_out_simu : Inport  Port=5
  inport-mot2_plant_temp_coeff_simu : Inport  Port=6
  Ground_1 : Ground
  Toworkspace-mot2_plant_cmd_simu : ToWorkspace  VariableName=mot2_plant_cmd_simu  SampleTime=pxf_diagram_options.workspace_sample_time
      settings: Decimation=pxf_diagram_options.decimation
  Toworkspace-mot2_plant_curr_in_simu : ToWorkspace  VariableName=mot2_plant_curr_in_simu  SampleTime=pxf_diagram_options.workspace_sample_time
      settings: Decimation=pxf_diagram_options.decimation
  Toworkspace-mot2_plant_spd_out_simu : ToWorkspace  VariableName=mot2_plant_spd_out_simu  SampleTime=pxf_diagram_options.workspace_sample_time
      settings: Decimation=pxf_diagram_options.decimation
  Toworkspace-mot2_plant_temp_coeff_simu : ToWorkspace  VariableName=mot2_plant_temp_coeff_simu  SampleTime=pxf_diagram_options.workspace_sample_time
      settings: Decimation=pxf_diagram_options.decimation
  Toworkspace-mot2_plant_trq_out_simu : ToWorkspace  VariableName=mot2_plant_trq_out_simu  SampleTime=pxf_diagram_options.workspace_sample_time
      settings: Decimation=pxf_diagram_options.decimation
  Toworkspace-mot2_plant_volt_in_simu : ToWorkspace  VariableName=mot2_plant_volt_in_simu  SampleTime=pxf_diagram_options.workspace_sample_time
      settings: Decimation=pxf_diagram_options.decimation
  create_system_info_bus : BusCreator  Inputs=2
  outport-system_info_bus : Outport
  outport-plant_bus : Outport  Port=2
  wires:
  create_system_info_bus/1 -> outport-system_info_bus/1
  inport-mot2_plant_spd_out_simu/1 -> create_system_info_bus/1, Toworkspace-mot2_plant_spd_out_simu/1  "mot2_plant_spd_out_simu"
  inport-mot2_plant_curr_in_simu/1 -> Toworkspace-mot2_plant_curr_in_simu/1
  inport-mot2_plant_volt_in_simu/1 -> Toworkspace-mot2_plant_volt_in_simu/1
  inport-mot2_plant_cmd_simu/1 -> Toworkspace-mot2_plant_cmd_simu/1
  inport-mot2_plant_trq_out_simu/1 -> Toworkspace-mot2_plant_trq_out_simu/1
  inport-mot2_plant_temp_coeff_simu/1 -> create_system_info_bus/2, Toworkspace-mot2_plant_temp_coeff_simu/1  "mot2_plant_temp_coeff_simu"
  Ground_1/1 -> outport-plant_bus/1

== system PowerSystemRef/powerplant/mot2/plant/parameter_selection ==
  Inport_1 : Inport
  inport-ctrl_bus-2 : Inport  Port=2
  Terminator_1 : Terminator
  select_ctrl_bus : BusSelector  OutputSignals=mot2_ctrl_cmd_simu
  outport-mot2_ctrl_cmd_simu-1 : Outport
  wires:
  inport-ctrl_bus-2/1 -> select_ctrl_bus/1
  select_ctrl_bus/1 -> outport-mot2_ctrl_cmd_simu-1/1  "<mot2_ctrl_cmd_simu>"
  Inport_1/1 -> Terminator_1/1

== system PowerSystemRef/powerplant/mot3/ctrl/cmd ==
  inport-main_info_bus-1 : Inport
  aInport--2 : Inport  Port=2
  aInport--3 : Inport  Port=3
  aInport--4 : Inport  Port=4
  Terminator_1 : Terminator
  Terminator_2 : Terminator
  Terminator_3 : Terminator
  mot3_ctrl_cmd_map_Pelec_funTW_volt_in : Subsystem
  parameter_out : Subsystem
  parameter_selection : Subsystem
  outport-system_info_bus : Outport
  wires:
  inport-main_info_bus-1/1 -> parameter_selection/1(inport-main_info_bus-1)
  parameter_out/1(outport-system_info_bus) -> outport-system_info_bus/1
  mot3_ctrl_cmd_map_Pelec_funTW_volt_in/1(mot_ctrl_cmd_simu) -> parameter_out/1(inport-mot3_ctrl_cmd_simu)
  parameter_selection/1(outport-mot3_plant_spd_out_simu-1) -> mot3_ctrl_cmd_map_Pelec_funTW_volt_in/1(mot_plant_spd_out_simu)
  parameter_selection/2(outport-mot3_ctrl_trs_trq_simu-2) -> mot3_ctrl_cmd_map_Pelec_funTW_volt_in/2(mot_ctrl_trs_trq_simu)
  parameter_selection/3(outport-mot3_ctrl_cstr_trq_max_pos_simu-3) -> mot3_ctrl_cmd_map_Pelec_funTW_volt_in/3(mot_ctrl_cstr_trq_max_pos_simu)
  parameter_selection/4(outport-mot3_ctrl_cstr_trq_max_neg_simu-4) -> mot3_ctrl_cmd_map_Pelec_funTW_volt_in/4(mot_ctrl_cstr_trq_max_neg_simu)
  aInport--2/1 -> Terminator_1/1
  aInport--3/1 -> Terminator_2/1
  aInport--4/1 -> Terminator_3/1

== system PowerSystemRef/powerplant/mot3/ctrl/cstr ==
  inport-main_info_bus-1 : Inport
  aInport--2 : Inport  Port=2
  aInport--3 : Inport  Port=3
  Terminator_1 : Terminator
  Terminator_2 : Terminator
  mot3_ctrl_cstr_map_Pelec_funTW_volt_in : Subsystem
  parameter_out : Subsystem
  parameter_selection : Subsystem
  outport-system_info_bus : Outport
  outport-cstr_bus : Outport  Port=2
  wires:
  inport-main_info_bus-1/1 -> parameter_selection/1(inport-main_info_bus-1)
  parameter_out/1(outport-system_info_bus) -> outport-system_info_bus/1
  parameter_out/2(outport-cstr_bus) -> outport-cstr_bus/1
  mot3_ctrl_cstr_map_Pelec_funTW_volt_in/1(mot_ctrl_cstr_trq_pk_pos_simu) -> parameter_out/1(inport-mot3_ctrl_cstr_trq_pk_pos_simu)
  mot3_ctrl_cstr_map_Pelec_funTW_volt_in/2(mot_ctrl_cstr_trq_max_pos_simu) -> parameter_out/2(inport-mot3_ctrl_cstr_trq_max_pos_simu)
  mot3_ctrl_cstr_map_Pelec_funTW_volt_in/3(mot_ctrl_cstr_trq_pk_neg_simu) -> parameter_out/3(inport-mot3_ctrl_cstr_trq_pk_neg_simu)
  mot3_ctrl_cstr_map_Pelec_funTW_volt_in/4(mot_ctrl_cstr_trq_max_neg_simu) -> parameter_out/4(inport-mot3_ctrl_cstr_trq_max_neg_simu)
  mot3_ctrl_cstr_map_Pelec_funTW_volt_in/5(mot_ctrl_cstr_trq_cont_pos_simu) -> parameter_out/5(inport-mot3_ctrl_cstr_trq_cont_pos_simu)
  mot3_ctrl_cstr_map_Pelec_funTW_volt_in/6(mot_ctrl_cstr_trq_cont_neg_simu) -> parameter_out/6(inport-mot3_ctrl_cstr_trq_cont_neg_simu)
  mot3_ctrl_cstr_map_Pelec_funTW_volt_in/7(mot_ctrl_cstr_temp_coeff_simu) -> parameter_out/7(inport-mot3_ctrl_cstr_temp_coeff_simu)
  parameter_selection/1(outport-mot3_plant_spd_out_simu-1) -> mot3_ctrl_cstr_map_Pelec_funTW_volt_in/1(mot_plant_spd_out_simu)
  parameter_selection/2(outport-mot3_plant_temp_coeff_simu-2) -> mot3_ctrl_cstr_map_Pelec_funTW_volt_in/2(mot_plant_temp_coeff_simu)
  aInport--2/1 -> Terminator_1/1
  aInport--3/1 -> Terminator_2/1

== system PowerSystemRef/powerplant/mot3/ctrl/dmd ==
  inport-main_info_bus-1 : Inport
  aInport--2 : Inport  Port=2
  Terminator_1 : Terminator
  mot3_ctrl_dmd_uas : Subsystem
  parameter_out : Subsystem
  parameter_selection : Subsystem
  outport-system_info_bus : Outport
  outport-dmd_bus : Outport  Port=2
  wires:
  inport-main_info_bus-1/1 -> parameter_selection/1(inport-main_info_bus-1)
  parameter_out/1(outport-system_info_bus) -> outport-system_info_bus/1
  parameter_out/2(outport-dmd_bus) -> outport-dmd_bus/1
  mot3_ctrl_dmd_uas/1(mot_ctrl_trs_trq_simu) -> parameter_out/1(inport-mot3_ctrl_trs_trq_simu)
  mot3_ctrl_dmd_uas/2(mot_ctrl_ratedpwr_simu) -> parameter_out/2(inport-mot3_ctrl_ratedpwr_simu)
  parameter_selection/1(outport-apc_ctrl_dt3_simu-1) -> mot3_ctrl_dmd_uas/1(apc_ctrl_dt_simu)
  parameter_selection/2(outport-env_plant_density_simu-2) -> mot3_ctrl_dmd_uas/2(env_plant_density_simu)
  parameter_selection/3(outport-ess_ctrl_pwr_max_pro_simu-3) -> mot3_ctrl_dmd_uas/3(ess_ctrl_pwr_max_pro_simu)
  parameter_selection/4(outport-propel3_plant_speed_simu-4) -> mot3_ctrl_dmd_uas/4(propel_plant_speed_simu)
  parameter_selection/5(outport-tc3_plant_spd_in_simu-5) -> mot3_ctrl_dmd_uas/5(tc_plant_spd_in_simu)
  aInport--2/1 -> Terminator_1/1

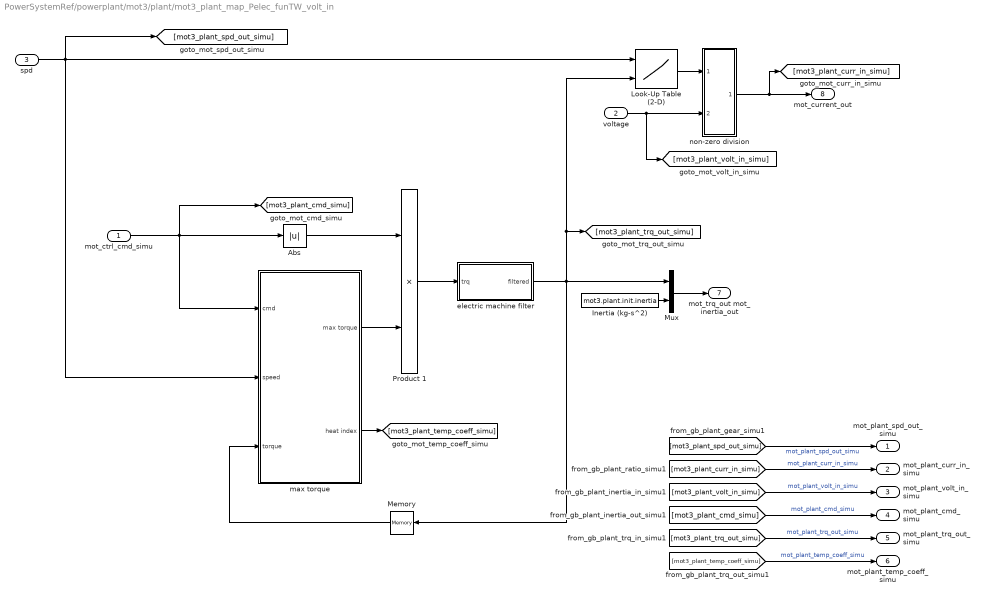
== system PowerSystemRef/powerplant/mot3/plant/mot3_plant_map_Pelec_funTW_volt_in ==
  mot_ctrl_cmd_simu : Inport
  voltage : Inport  Port=2
  spd : Inport  Port=3
  Abs : Abs
  Inertia (kg-s^2) : Constant  Value=mot3.plant.init.inertia
  Look-Up Table (2-D) : Lookup2D  RowIndex=mot3.plant.calc.pwr_elec.idx1_spd  ColumnIndex=mot3.plant.calc.pwr_elec.idx2_trq  Table=mot3.plant.calc.pwr_elec.map
  Memory : Memory
  Mux : Mux  Inputs=2
  Product 1 : Product  InputSameDT=on  SaturateOnIntegerOverflow=on  OutDataTypeStr=Inherit: Same as first input
  electric machine filter : Subsystem
  "max torque " : Subsystem
  non-zero division : Subsystem
      mask Display: disp('divider \n I1/I2')
  mot_plant_spd_out_simu : Outport
  mot_plant_curr_in_simu : Outport  Port=2
  mot_plant_volt_in_simu : Outport  Port=3
  mot_plant_cmd_simu : Outport  Port=4
  mot_plant_trq_out_simu : Outport  Port=5
  mot_plant_temp_coeff_simu : Outport  Port=6
  mot_trq_out mot_inertia_out : Outport  Port=7
  mot_current_out : Outport  Port=8
  wires:
  Look-Up Table (2-D)/1 -> non-zero division/1(In1)
  [mot3_plant_temp_coeff_simu] -> mot_plant_temp_coeff_simu/1  "mot_plant_temp_coeff_simu"
  [mot3_plant_trq_out_simu] -> mot_plant_trq_out_simu/1  "mot_plant_trq_out_simu"
  [mot3_plant_cmd_simu] -> mot_plant_cmd_simu/1  "mot_plant_cmd_simu"
  [mot3_plant_volt_in_simu] -> mot_plant_volt_in_simu/1  "mot_plant_volt_in_simu"
  [mot3_plant_curr_in_simu] -> mot_plant_curr_in_simu/1  "mot_plant_curr_in_simu"
  [mot3_plant_spd_out_simu] -> mot_plant_spd_out_simu/1  "mot_plant_spd_out_simu"
  electric machine filter/1(filtered) -> Mux/1, Memory/1, [mot3_plant_trq_out_simu], Look-Up Table (2-D)/2
  "max torque "/1(max torque) -> Product 1/2
  Product 1/1 -> electric machine filter/1(trq)
  Abs/1 -> Product 1/1
  Memory/1 -> "max torque "/3(torque)
  mot_ctrl_cmd_simu/1 -> "max torque "/1(cmd), [mot3_plant_cmd_simu], Abs/1
  Inertia (kg-s^2)/1 -> Mux/2
  Mux/1 -> mot_trq_out mot_inertia_out/1
  spd/1 -> [mot3_plant_spd_out_simu], "max torque "/2(speed), Look-Up Table (2-D)/1
  "max torque "/2(heat index) -> [mot3_plant_temp_coeff_simu]
  non-zero division/1(Out1) -> mot_current_out/1, [mot3_plant_curr_in_simu]
  voltage/1 -> non-zero division/2(In2), [mot3_plant_volt_in_simu]

== system PowerSystemRef/powerplant/mot3/plant/parameter_out ==
  inport-mot3_plant_spd_out_simu : Inport
  inport-mot3_plant_curr_in_simu : Inport  Port=2
  inport-mot3_plant_volt_in_simu : Inport  Port=3
  inport-mot3_plant_cmd_simu : Inport  Port=4
  inport-mot3_plant_trq_out_simu : Inport  Port=5
  inport-mot3_plant_temp_coeff_simu : Inport  Port=6
  Ground_1 : Ground
  Toworkspace-mot3_plant_cmd_simu : ToWorkspace  VariableName=mot3_plant_cmd_simu  SampleTime=pxf_diagram_options.workspace_sample_time
      settings: Decimation=pxf_diagram_options.decimation
  Toworkspace-mot3_plant_curr_in_simu : ToWorkspace  VariableName=mot3_plant_curr_in_simu  SampleTime=pxf_diagram_options.workspace_sample_time
      settings: Decimation=pxf_diagram_options.decimation
  Toworkspace-mot3_plant_spd_out_simu : ToWorkspace  VariableName=mot3_plant_spd_out_simu  SampleTime=pxf_diagram_options.workspace_sample_time
      settings: Decimation=pxf_diagram_options.decimation
  Toworkspace-mot3_plant_temp_coeff_simu : ToWorkspace  VariableName=mot3_plant_temp_coeff_simu  SampleTime=pxf_diagram_options.workspace_sample_time
      settings: Decimation=pxf_diagram_options.decimation
  Toworkspace-mot3_plant_trq_out_simu : ToWorkspace  VariableName=mot3_plant_trq_out_simu  SampleTime=pxf_diagram_options.workspace_sample_time
      settings: Decimation=pxf_diagram_options.decimation
  Toworkspace-mot3_plant_volt_in_simu : ToWorkspace  VariableName=mot3_plant_volt_in_simu  SampleTime=pxf_diagram_options.workspace_sample_time
      settings: Decimation=pxf_diagram_options.decimation
  create_system_info_bus : BusCreator  Inputs=2
  outport-system_info_bus : Outport
  outport-plant_bus : Outport  Port=2
  wires:
  create_system_info_bus/1 -> outport-system_info_bus/1
  inport-mot3_plant_spd_out_simu/1 -> create_system_info_bus/1, Toworkspace-mot3_plant_spd_out_simu/1  "mot3_plant_spd_out_simu"
  inport-mot3_plant_curr_in_simu/1 -> Toworkspace-mot3_plant_curr_in_simu/1
  inport-mot3_plant_volt_in_simu/1 -> Toworkspace-mot3_plant_volt_in_simu/1
  inport-mot3_plant_cmd_simu/1 -> Toworkspace-mot3_plant_cmd_simu/1
  inport-mot3_plant_trq_out_simu/1 -> Toworkspace-mot3_plant_trq_out_simu/1
  inport-mot3_plant_temp_coeff_simu/1 -> create_system_info_bus/2, Toworkspace-mot3_plant_temp_coeff_simu/1  "mot3_plant_temp_coeff_simu"
  Ground_1/1 -> outport-plant_bus/1

== system PowerSystemRef/powerplant/mot3/plant/parameter_selection ==
  Inport_1 : Inport
  inport-ctrl_bus-2 : Inport  Port=2
  Terminator_1 : Terminator
  select_ctrl_bus : BusSelector  OutputSignals=mot3_ctrl_cmd_simu
  outport-mot3_ctrl_cmd_simu-1 : Outport
  wires:
  inport-ctrl_bus-2/1 -> select_ctrl_bus/1
  select_ctrl_bus/1 -> outport-mot3_ctrl_cmd_simu-1/1  "<mot3_ctrl_cmd_simu>"
  Inport_1/1 -> Terminator_1/1
